simulink model "sf_angle_events"  (R2017b)
settings: Solver=VariableStepAuto  StartTime=0.0  StopTime=20  MaxStep=inf  RelTol=1e-6  EnableMultiTasking=on
StopFcn:
  | %dt = [diff(tout); nan];
  | %plot(tout, dt, '.'); grid;
  | %title('Step size is driven by crank angle events');
  | %ylabel('Step size');
  | %xlabel('Time');
undefined symbols (not defined in the file): setdiff
libraries: simulink x1
settings Model: Creator=The MathWorks, Inc.  LastModifiedBy=The MathWorks, Inc.
settings DataIOCC: SaveOutput=off
settings OptimizationCC: LifeSpan=inf
settings DebuggingCC: AllowSymbolicDim=off  SFUnexpectedBacktrackingDiag=warning  SFNoUnconditionalDefaultTransitionDiag=warning  SFExecutionAtInitializationDiag=none
settings ModelReferenceCC: PropagateSignalLabelsOutOfModel=off
settings CodeAppCC: StateflowObjectComments=on
settings GRTTargetCC: TargetLangStandard=C89/C90 (ANSI)
settings ConfigComp: CovMetricSettings=dw  CovHtmlReporting=on  CovSaveCumulativeToWorkspaceVar=on  CovSaveSingleToWorkspaceVar=on  CovExternalEMLEnable=off

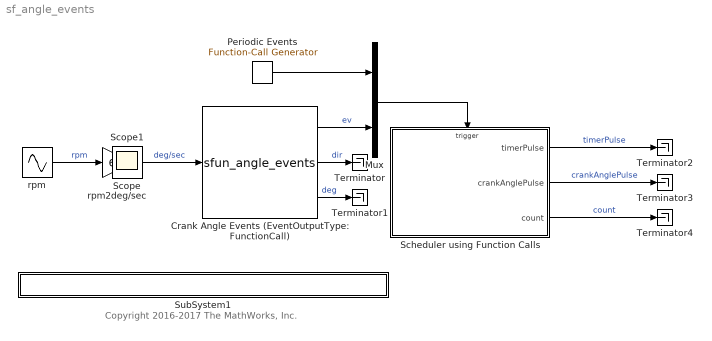
== system sf_angle_events ==
  note: Copyright 2016-2017 The MathWorks, Inc.
  Crank Angle Events (EventOutputType: FunctionCall) : S-Function  LoadFcn=|  FunctionName=sfun_angle_events  Parameters=CrossingAngles, InitialAngle, eventOutputType, clockwiseOnly  SFunctionDeploymentMode=off  EnableBusSupport=off  mask(AnglularIntegratorWithEventDetection){CrossingAngles=setdiff([0:6:354],[120 126]), InitialAngle=0, EventOutputType=Function Call, ClockwiseOnly=on}
      | DVG.Registry.registerIcon(...
      | 'BlockIcon.SFunAngleEvents', ...
      | fullfile(matlabroot,'toolbox','simulink','simdemos','simfeatures','slexToothedWheel.svg'))
      mask prompts: CrossingAngles "Crossing Angles:"; InitialAngle "Initial Angle:"; EventOutputType "Event output type:"; ClockwiseOnly "Assume clockwise rotation only"
      mask help:
      | This block integrates the angular velocity input to compute the angle and to fire events at the specified crossing angles. All angles are in degrees, with 0 at the top, incresing clockwise.
      |
      | The crossings angles should be specified as a monotonically increasing vector, with the first element set to 0 and the last element being less than 360 degrees.
      |
      | The first output is a function call, which is fired when an angle crossing event is detected.
      |
      | The second output indicates the direction of the angle crossing event, true for clockwise and false for anti-clockwise.
      |
      | The third output is the angle, wrapped to be in [0, 360) degrees.
      mask init:
      | clockwiseOnly = isequal(get_param(gcb,'ClockwiseOnly'),'on');
      | 
      | switch get_param(gcb,'EventOutputType')
      |     case 'Trigger Pulse'
      |         eventOutputType = 0;
      |     case 'Function Call'
      |         eventOutputType = 1;
      |     otherwise
      |         eventOutputType = 2;
      | end
      mask TypeOptions EventOutputType: Trigger Pulse | Function Call
      mask Display: %image('slexToothedWheel.svg');
  Mux : Mux  Inputs=2
  Periodic Events : simulink/Ports & Subsystems/Function-Call Generator  sample_time=0.001  numberOfIterations=1
      settings: AttributesFormatString=[Period=%<sample_time>]
  Scheduler using Function Calls : Stateflow chart  TreatAsAtomicUnit=on
  SubSystem1 : Subsystem  mask{filename=sfun_angle_events.c}
      mask init:
      | x=sfundemo_maskdisp;
      settings: AttributesFormatString=\n  OpenFcn=sfundemo_openfcn
      mask Display: disp(x);
  Terminator{,1..4} (5 alike) : Terminator
  rpm : Sin  Amplitude=2700  Bias=3300  Frequency=pi/5  SampleTime=0
  rpm2deg/sec : Gain  Gain=6
  Scope : Scope
  Scope1 : Scope
  wires:
  Crank Angle Events (EventOutputType: FunctionCall)/1 -> Mux/2  "ev"
  rpm/1 -> rpm2deg/sec/1  "rpm"
  rpm2deg/sec/1 -> Crank Angle Events (EventOutputType: FunctionCall)/1  "deg/sec"
  Crank Angle Events (EventOutputType: FunctionCall)/2 -> Terminator/1  "dir"
  Periodic Events/1 -> Mux/1
  Crank Angle Events (EventOutputType: FunctionCall)/3 -> Terminator1/1  "deg"
  Mux/1 -> Scheduler using Function Calls/Trigger
  Scheduler using Function Calls/1(timerPulse) -> Terminator2/1  "timerPulse"
  Scheduler using Function Calls/2(crankAnglePulse) -> Terminator3/1  "crankAnglePulse"
  Scheduler using Function Calls/3(count) -> Terminator4/1  "count"

== system sf_angle_events/SubSystem1 ==

== stateflow chart sf_angle_events/Scheduler using Function Calls ==
  state DefaultState
  (default) -> DefaultState
  DefaultState -> (junction 14)
  (junction 14) -> (junction 9)
  (junction 9) -> DefaultState [order 1] : [crankAngleEvent]
      |
      | {crankAnglePulse = ~crankAnglePulse;
      | count = count+1;}
  (junction 9) -> (junction 10) [order 2]
  (junction 10) -> DefaultState : [timerEvent]
      |
      | {timerPulse = ~timerPulse;
      | count = 0;}
  data: timerPulse output boolean size=1 =false; crankAnglePulse output boolean size=1 =false; count output uint32 =uint32(0)
  events: timerEvent input FUNCTION_CALL_EVENT; crankAngleEvent input FUNCTION_CALL_EVENT
